simulink model "Fig_11_12_13_"  (R2024a)
settings: Solver=VariableStepAuto  StartTime=0.0  StopTime=1  RelTol=1e-3
undefined symbols (not defined in the file): gcbh, Ion, Lithium, sps_rtmsupport
libraries: spsSeriesRLCBranchLib x11, slpidlib x5, spsIGBTDiodeLib x4, spsVoltageMeasurementLib x4, spsThreePhaseVIMeasurementLib x4, spsThreePhaseSeriesRLCBranchLib x4, spsUniversalBridgeLib x3, spsPWMGeneratorDCDCLib x3, spsVIMeasurementModel x3, spsDiodeLib x2, spsabctodq0Lib x2, spsCurrentMeasurementLib x2
(part 1 of 2)
settings Model: Creator=MS  LastModifiedBy=Dileep Uppara
settings DataIOCC: ReturnWorkspaceOutputs=off

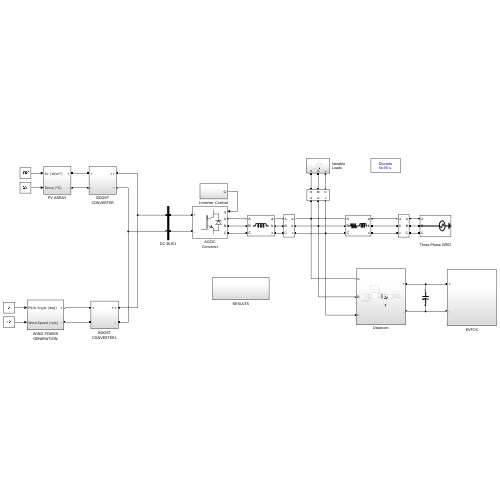
[thumbnail: Simulink's stored preview of the top-level diagram]
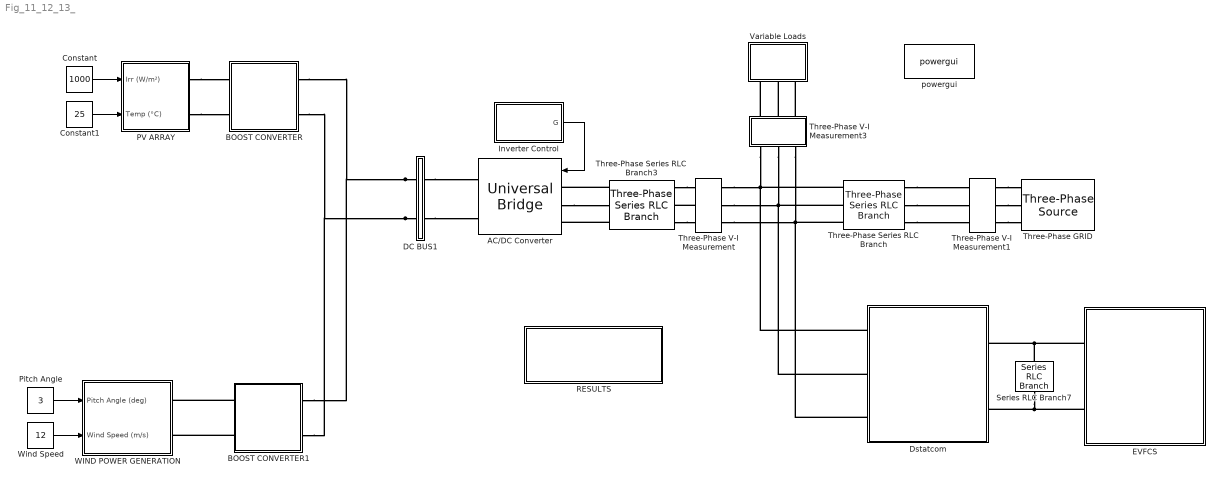
== system Fig_11_12_13_ ==
  " Three-Phase GRID" : spsThreePhaseSourceLib/Three-Phase Source  InternalConnection=Yg  VoltagePhases=off  Voltage=400  PhaseAngle=0  Voltage_phases=[25e3 25e3 25e3]/sqrt(3)  PhaseAngles_phases=[0 -120 +120]  Frequency=50  NonIdealSource=on  SpecifyImpedance=off  Resistance=0  Inductance=0  ShortCircuitLevel=100e6  BaseVoltage=0  XRratio=7  BusType=swing  Pref=0  Qref=0  Prefabc=[10e3, 10e3, 10e3]  Qrefabc=[0, 0, 0]  Qmin=-inf  Qmax=inf
  AC/DC Converter : spsUniversalBridgeLib/Universal Bridge  Arms=3  SnubberResistance=1e5  SnubberCapacitance=inf  Device=IGBT / Diodes  Ron=1e-3  Lon=0  ForwardVoltages="[  0  0  ]"  ForwardVoltage=0  GTOparameters=[ 10e-6 , 20e-6 ]  IGBTparameters=[ 1e-6 , 2e-6 ]  Measurements=None  Measurements_2=None  converterType=Rectifier
  BOOST CONVERTER : Subsystem
  BOOST CONVERTER1 : Subsystem
  Constant : Constant  Value=1000  SampleTime=50e-6
  Constant1 : Constant  Value=25  SampleTime=50e-6
  DC BUS1 : Subsystem
  Dstatcom : Subsystem
  EVFCS : Subsystem
  Inverter Control : Subsystem
  PV ARRAY : Subsystem
  "Pitch Angle " : Constant  Value=3  SampleTime=50e-6
  RESULTS : Subsystem
  Series RLC Branch7 : spsSeriesRLCBranchLib/Series RLC Branch  LConnTagsString=__new0  RConnTagsString=__new0  BranchType=C  Resistance=1  Inductance=1e-3  SetiL0=off  InitialCurrent=0  Capacitance=1000e-6  Setx0=on  InitialVoltage=800  Measurements=None
  Three-Phase Series RLC Branch : spsThreePhaseSeriesRLCBranchLib/Three-Phase Series RLC Branch  LConnTagsString=A|B|C  RConnTagsString=A|B|C  BranchType=RL  Resistance=2.088  Inductance=0.01e-3  Capacitance=1e-6  Measurements=None
  Three-Phase Series RLC Branch3 : spsThreePhaseSeriesRLCBranchLib/Three-Phase Series RLC Branch  LConnTagsString=A|B|C  RConnTagsString=A|B|C  BranchType=L  Resistance=3  Inductance=20e-3  Capacitance=1e-6  Measurements=None
  Three-Phase V-I Measurement : spsThreePhaseVIMeasurementLib/Three-Phase V-I Measurement  VoltageMeasurement=phase-to-ground  SetLabelV=on  LabelV=Viabc  Vpu=off  VpuLL=off  CurrentMeasurement=yes  SetLabelI=on  LabelI=Iiabc  Ipu=off  Pbase=100e6  Vbase=500e3  OutputType=Complex  PhasorSimulation=off  PSBequivalent=0
  Three-Phase V-I Measurement1 : spsThreePhaseVIMeasurementLib/Three-Phase V-I Measurement  VoltageMeasurement=phase-to-ground  SetLabelV=on  LabelV=Vgabc  Vpu=off  VpuLL=off  CurrentMeasurement=yes  SetLabelI=on  LabelI=Igabc  Ipu=off  Pbase=100e6  Vbase=500e3  OutputType=Complex  PhasorSimulation=off  PSBequivalent=0
  Three-Phase V-I Measurement3 : Subsystem  DialogController=POWERSYS.PowerSysDialog  LoadFcn=|  StartFcn=sps_rtmsupport('StartFcn',gcbh);  StopFcn=sps_rtmsupport('StopFcn',gcbh);  mask(Three-Phase VI Measurement){VoltageMeasurement=phase-to-ground, SetLabelV=on, LabelV=Vlabc, Vpu=off, VpuLL=off, CurrentMeasurement=yes, SetLabelI=on, LabelI=Ilabc, Ipu=off, Pbase=100e6, Vbase=500e3, OutputType=Complex, PhasorSimulation=off, PSBequivalent=0}
      | if ~strcmp(get_param(bdroot,'BlockDiagramType'),'library')
      |     set_param([gcb,'/Model'],'LinkStatus','restore');
      | end
      | sps_rtmsupport('LoadFcn',gcbh);
      mask prompts: VoltageMeasurement "Voltage measurement"; SetLabelV "Use a label"; LabelV "Signal label  (use a From block to collect this signal)"; Vpu "Voltages in pu,  based on peak value of nominal phase-to-ground voltage"; VpuLL "Voltages in pu,  based on peak value of nominal phase-to-phase  voltage"; CurrentMeasurement "Current measurement"; SetLabelI "Use a label"; LabelI "Signal label  (use a From block to collect this signal)"; Ipu "Currents in pu"; Pbase "Base power ( VA 3 phase)"; Vbase "Nominal voltage used for pu measurement (Vrms phase-phase) :"; OutputType "Output signals in:"; PhasorSimulation "Phasor simulation (internal use)"; PSBequivalent "Equivalent circuit (internal use)"
      mask help:
      | Ideal three-phase voltage and current measurements.
      |
      | The block can output the voltages and currents in per unit values or in volts and amperes.
      mask init:
      | block = gcb;
      | Kv=1;
      | Ki=1;
      | [Kv,Ki] = powericon('ThreePhaseVIMeasurementParam',block,Vpu,VpuLL,Ipu,Vbase,Pbase,PhasorSimulation,OutputType);
      | powericon('ThreePhaseVIMeasurementCback',block);
      | power_initmask();
      settings: CopyFcn=sps_rtmsupport('CopyFcn',gcbh); powericon('ThreePhaseVIMeasurementCopy',gcb)  DeleteFcn=sps_rtmsupport('DeleteFcn',gcbh);  UndoDeleteFcn=sps_rtmsupport('UndoDeleteFcn',gcbh);  ModelCloseFcn=sps_rtmsupport('ModelCloseFcn',gcbh);  PostSaveFcn=sps_rtmsupport('PostSaveFcn',gcbh);  NameChangeFcn=sps_rtmsupport('NameChangeFcn',gcbh);  PreCopyFcn=sps_rtmsupport('PreCopyFcn',gcbh);  OpenFcn=sps_rtmsupport('OpenFcn',gcbh, [1 2 4 5 6 7 9 -12 13]);  CloseFcn=sps_rtmsupport('CloseFcn',gcbh);  PreDeleteFcn=sps_rtmsupport('PreDeleteFcn',gcbh);
      settings: LibrarySourceBlock=|
      | sps_lib/Sensors and Measurements/Three-Phase
      | V-I Measurement
      settings: PreSaveFcn=|
      | sps_rtmsupport('PreSaveFcn',gcbh);
      | if ~strcmp(get_param(bdroot(gcbh),'BlockDiagramType'),'library')
      |     set_param(gcb,'LinkStatus','restore')
      | end
      mask Help: helpview(psbhelp)
      mask TypeOptions VoltageMeasurement: no | phase-to-ground | phase-to-phase
      mask Callback VoltageMeasurement: powericon('ThreePhaseVIMeasurementCback',gcb,'Vselector');
      mask Callback SetLabelV: powericon('ThreePhaseVIMeasurementCback',gcb,'');
      mask Callback Vpu: powericon('ThreePhaseVIMeasurementCback',gcb,'Vpu');
      mask Callback VpuLL: powericon('ThreePhaseVIMeasurementCback',gcb,'VpuLL');
      mask TypeOptions CurrentMeasurement: no | yes
      mask Callback CurrentMeasurement: powericon('ThreePhaseVIMeasurementCback',gcb,'');
      mask Callback SetLabelI: powericon('ThreePhaseVIMeasurementCback',gcb,'');
      mask Callback LabelI: powericon('ThreePhaseVIMeasurementCback',gcb,'');
      mask Callback Ipu: powericon('ThreePhaseVIMeasurementCback',gcb,'');
      mask TypeOptions OutputType: Complex | Real-Imag | Magnitude-Angle | Magnitude
  Variable Loads : Subsystem
  WIND POWER GENERATION : Subsystem
  Wind Speed : Constant  Value=12  SampleTime=50e-6
  powergui : spspowerguiLib/powergui  Priority=1  SimulationMode=Discrete  SampleTime=50e-6  frequency=60  Iterations=50  frequencyindice=0  Pbase=100e6  ErrMax=1e-4  UnitsV=kV  UnitsW=MW  buscounter=0  FunctionMessages=off  echomessages=off  EnableUseOfTLC=off  CurrentSourceSwitches=off  DisableSnubberDevices=off  DisableRonSwitches=off  DisableVfSwitches=off  DisplayEquations=off  AutomaticDiscreteSolvers=off  SolverType=Tustin/Backward Euler (TBE)  Interpol=off  ExternalGateDelay=off  methode=off  Ts=100  x0status=blocks  SPID=on  SwTol=0  HookPort=off  NonlinearTolerance=1e-4  nMaxIteration=100  ContinueOnMaxIteration=off  RestoreLinks=warning  ResistiveCurrentMeasurement=off  Frange=[0:2:500]  Ylog=off  Xlog=on  ShowGrid=off  save=off  variable=ZData  structure=0  ZoomFFT=off  StartTime=0.0  cycles=1  DisplayStyle=1  fundamental=60  FreqAxis=off  MaxFrequency=1000  frequencyindicesteady=1  RmsSteady=1  display=off
  wires:
  Inverter Control/1(G) -> AC/DC Converter/1
  Wind Speed/1 -> WIND POWER GENERATION/2(Wind Speed (m/s))
  "Pitch Angle "/1 -> WIND POWER GENERATION/1(Pitch Angle (deg))
  Constant/1 -> PV ARRAY/1(Irr (W/m²))
  Constant1/1 -> PV ARRAY/2(Temp (°C))
  connections:
  Three-Phase Series RLC Branch3/LConn1 -- AC/DC Converter/LConn1
  AC/DC Converter/LConn2 -- Three-Phase Series RLC Branch3/LConn2
  Three-Phase Series RLC Branch3/LConn3 -- AC/DC Converter/LConn3
  Three-Phase Series RLC Branch3/RConn1 -- Three-Phase V-I Measurement/LConn1
  Three-Phase V-I Measurement/LConn2 -- Three-Phase Series RLC Branch3/RConn2
  Three-Phase Series RLC Branch3/RConn3 -- Three-Phase V-I Measurement/LConn3
  DC BUS1/RConn2 -- AC/DC Converter/RConn2
  DC BUS1/RConn1 -- AC/DC Converter/RConn1
  Three-Phase V-I Measurement/RConn1 -- Three-Phase V-I Measurement3/RConn1 -- Three-Phase Series RLC Branch/LConn1 -- Dstatcom/RConn1
  Three-Phase V-I Measurement/RConn3 -- Three-Phase V-I Measurement3/RConn3 -- Three-Phase Series RLC Branch/LConn3 -- Dstatcom/RConn3
  Three-Phase V-I Measurement/RConn2 -- Three-Phase V-I Measurement3/RConn2 -- Three-Phase Series RLC Branch/LConn2 -- Dstatcom/RConn2
  Series RLC Branch7/LConn1 -- EVFCS/RConn1 -- Dstatcom/LConn1
  Series RLC Branch7/RConn1 -- Dstatcom/LConn2 -- EVFCS/RConn2
  DC BUS1/LConn2 -- BOOST CONVERTER/RConn2 -- BOOST CONVERTER1/RConn2
  DC BUS1/LConn1 -- BOOST CONVERTER/RConn1 -- BOOST CONVERTER1/RConn1
  Three-Phase V-I Measurement3/LConn2 -- Variable Loads/LConn2
  Three-Phase V-I Measurement3/LConn1 -- Variable Loads/LConn1
  Three-Phase V-I Measurement3/LConn3 -- Variable Loads/LConn3
  PV ARRAY/RConn1 -- BOOST CONVERTER/LConn1
  PV ARRAY/RConn2 -- BOOST CONVERTER/LConn2
  BOOST CONVERTER1/LConn2 -- WIND POWER GENERATION/RConn2
  BOOST CONVERTER1/LConn1 -- WIND POWER GENERATION/RConn1
  Three-Phase V-I Measurement1/LConn1 -- " Three-Phase GRID"/RConn1
  Three-Phase Series RLC Branch/RConn2 -- Three-Phase V-I Measurement1/RConn2
  Three-Phase V-I Measurement1/LConn3 -- " Three-Phase GRID"/RConn3
  Three-Phase Series RLC Branch/RConn1 -- Three-Phase V-I Measurement1/RConn1
  Three-Phase V-I Measurement1/LConn2 -- " Three-Phase GRID"/RConn2
  Three-Phase Series RLC Branch/RConn3 -- Three-Phase V-I Measurement1/RConn3

== system Fig_11_12_13_/BOOST CONVERTER ==
  Diode : spsDiodeLib/Diode  Ron=0.001  Lon=0  Vf=0.8  IC=0  UseSnubber=0  Rs=500  Cs=250e-9  Measurements=off
  IGBT/Diode : spsIGBTDiodeLib/IGBT//Diode  Ron=1e-3  Rs=1e5  Cs=inf  Measurements=off
  PWM Generator (DC-DC) : spsPWMGeneratorDCDCLib/PWM Generator (DC-DC)  Fsw=15e3  Ts=50e-6
  PnO : Subsystem
  Series RLC Branch : spsSeriesRLCBranchLib/Series RLC Branch  LConnTagsString=__new0  RConnTagsString=__new0  BranchType=L  Resistance=0.01  Inductance=0.009e-3  SetiL0=off  InitialCurrent=0  Capacitance=1e-6  Setx0=off  InitialVoltage=0  Measurements=None
  Series RLC Branch1 : spsSeriesRLCBranchLib/Series RLC Branch  LConnTagsString=__new0  RConnTagsString=__new0  BranchType=C  Resistance=0.01  Inductance=0.5e-3  SetiL0=off  InitialCurrent=0  Capacitance=880e-6  Setx0=off  InitialVoltage=0  Measurements=None
  Series RLC Branch2 : spsSeriesRLCBranchLib/Series RLC Branch  LConnTagsString=__new0  RConnTagsString=__new0  BranchType=C  Resistance=0.01  Inductance=0.5e-3  SetiL0=off  InitialCurrent=0  Capacitance=880e-6  Setx0=off  InitialVoltage=0  Measurements=None
  + : PMIOPort  Side=Left
  - : PMIOPort  Port=2  Side=Left
  ++ : PMIOPort  Port=3  Side=Right
  -- : PMIOPort  Port=4  Side=Right
  wires:
  PWM Generator (DC-DC)/1 -> IGBT/Diode/1
  PnO/1(D) -> PWM Generator (DC-DC)/1
  connections:
  Series RLC Branch/RConn1 -- Diode/LConn1 -- IGBT/Diode/LConn1
  +/RConn1 -- Series RLC Branch2/LConn1 -- Series RLC Branch/LConn1
  Series RLC Branch2/RConn1 -- -/RConn1 -- Series RLC Branch1/RConn1 -- --/RConn1 -- IGBT/Diode/RConn1
  Diode/RConn1 -- ++/RConn1 -- Series RLC Branch1/LConn1

== system Fig_11_12_13_/BOOST CONVERTER1 ==
  Diode : spsDiodeLib/Diode  Ron=0.001  Lon=0  Vf=0.8  IC=0  UseSnubber=0  Rs=500  Cs=250e-9  Measurements=off
  IGBT/Diode : spsIGBTDiodeLib/IGBT//Diode  Ron=1e-3  Rs=1e5  Cs=inf  Measurements=off
  PWM Generator (DC-DC) : spsPWMGeneratorDCDCLib/PWM Generator (DC-DC)  Fsw=15e3  Ts=50e-6
  PnO : Subsystem
  Series RLC Branch : spsSeriesRLCBranchLib/Series RLC Branch  LConnTagsString=__new0  RConnTagsString=__new0  BranchType=RL  Resistance=1.524  Inductance=0.1e-3  SetiL0=off  InitialCurrent=0  Capacitance=1e-6  Setx0=off  InitialVoltage=0  Measurements=None
  Series RLC Branch1 : spsSeriesRLCBranchLib/Series RLC Branch  LConnTagsString=__new0  RConnTagsString=__new0  BranchType=C  Resistance=0.01  Inductance=0.5e-3  SetiL0=off  InitialCurrent=0  Capacitance=880e-6  Setx0=off  InitialVoltage=0  Measurements=None
  + : PMIOPort  Side=Left
  - : PMIOPort  Port=2  Side=Left
  ++ : PMIOPort  Port=3  Side=Right
  -- : PMIOPort  Port=4  Side=Right
  wires:
  PWM Generator (DC-DC)/1 -> IGBT/Diode/1
  PnO/1(D) -> PWM Generator (DC-DC)/1
  connections:
  Series RLC Branch/RConn1 -- Diode/LConn1 -- IGBT/Diode/LConn1
  Diode/RConn1 -- Series RLC Branch1/LConn1 -- ++/RConn1
  +/RConn1 -- Series RLC Branch/LConn1
  -/RConn1 -- Series RLC Branch1/RConn1 -- --/RConn1 -- IGBT/Diode/RConn1

== system Fig_11_12_13_/DC BUS1 ==
  Display5 : Display
  Scope5 : Scope
  Series RLC Branch1 : spsSeriesRLCBranchLib/Series RLC Branch  LConnTagsString=__new0  RConnTagsString=__new0  BranchType=C  Resistance=0.01  Inductance=0.5e-3  SetiL0=off  InitialCurrent=0  Capacitance=10000e-6  Setx0=off  InitialVoltage=0  Measurements=None
  Voltage Measurement1 : spsVoltageMeasurementLib/Voltage Measurement  PhasorSimulation=off  OutputType=Complex  PSBequivalent=0
  ++ : PMIOPort  Side=Left
  Connection Port1 : PMIOPort  Port=2  Side=Left
  + : PMIOPort  Port=3  Side=Right
  - : PMIOPort  Port=4  Side=Right
  tag scope: Vdc=global
  wires:
  Voltage Measurement1/1 -> [Vdc], Display5/1, Scope5/1
  connections:
  -/RConn1 -- Voltage Measurement1/LConn2 -- Series RLC Branch1/RConn1 -- Connection Port1/RConn1
  +/RConn1 -- Series RLC Branch1/LConn1 -- ++/RConn1 -- Voltage Measurement1/LConn1

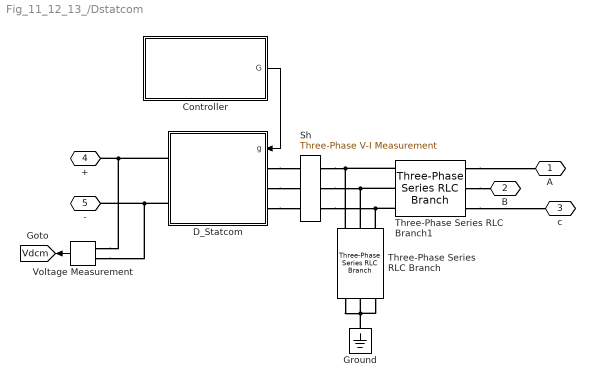
== system Fig_11_12_13_/Dstatcom ==
  Controller : Subsystem
  D_Statcom : Subsystem  DialogController=POWERSYS.PowerSysDialog  LoadFcn=sps_rtmsupport('LoadFcn',gcbh);  StartFcn=sps_rtmsupport('StartFcn',gcbh);  StopFcn=sps_rtmsupport('StopFcn',gcbh);  mask(Universal Bridge){Arms=3, SnubberResistance=1e5, SnubberCapacitance=inf, Device=IGBT / Diodes, Ron=1e-3, Lon=0, ForwardVoltages=[  0  0  ], ForwardVoltage=0, GTOparameters=[ 10e-6 , 20e-6 ], IGBTparameters=[ 1e-6 , 2e-6 ], Measurements=None, Measurements_2=None, converterType=Rectifier}
      mask prompts: Arms "Number of bridge arms:"; SnubberResistance "Snubber resistance Rs (Ohms)"; SnubberCapacitance "Snubber capacitance Cs (F)"; Device "Power Electronic device"; Ron "Ron (Ohms)"; Lon "Lon (H)"; ForwardVoltages "Forward voltages  [ Device Vf(V) , Diode Vfd(V)]"; ForwardVoltage "Forward voltage Vf (V)"; GTOparameters "[  Tf (s) , Tt (s)  ]"; IGBTparameters "[  Tf (s) , Tt (s)  ]"; Measurements_2 "Measurements"; converterType "Converter type:"
      mask help: This block implement a bridge of selected power electronics devices. Series RC snubber circuits are connected in parallel with each switch device. Press Help for suggested snubber values when the model is discretized. For most applications the internal inductance Lon of diodes and thyristors should be set to zero
      mask init:
      | block = gcb;
      | [WantBlockChoice,Ts,Switches,Tf_sps,Tt_sps,Vf,Vf_SwitchOn,Vf_DiodeOn,IC,SignalLength,ReorderGatesDelays,X,Y,Ron] = powericon('UniversalBridgeInit',block,Device,Arms,ForwardVoltage,ForwardVoltages,GTOparameters,IGBTparameters,Ron);
      | powericon('SetInternalModels','set',block,WantBlockChoice);
      settings: LibrarySourceBlock=sps_lib/Power Electronics/Universal Bridge  CopyFcn=sps_rtmsupport('CopyFcn',gcbh); powericon('SwitchesCopyFcn','Universal Bridge',gcb)  DeleteFcn=sps_rtmsupport('DeleteFcn',gcbh);  UndoDeleteFcn=sps_rtmsupport('UndoDeleteFcn',gcbh);  ModelCloseFcn=sps_rtmsupport('ModelCloseFcn',gcbh);  PreSaveFcn=sps_rtmsupport('PreSaveFcn',gcbh);  PostSaveFcn=sps_rtmsupport('PostSaveFcn',gcbh);  NameChangeFcn=sps_rtmsupport('NameChangeFcn',gcbh);  PreCopyFcn=sps_rtmsupport('PreCopyFcn',gcbh);  OpenFcn=sps_rtmsupport('OpenFcn',gcbh, [1 4 11 12 13]);  CloseFcn=sps_rtmsupport('CloseFcn',gcbh);  PreDeleteFcn=sps_rtmsupport('PreDeleteFcn',gcbh);
      mask Help: helpview(psbhelp);
      mask TypeOptions Arms: 1 | 2 | 3
      mask Callback Arms: powericon('UniversalBridgeCback',gcb);
      mask TypeOptions Device: Diodes | Thyristors | GTO / Diodes | MOSFET / Diodes | IGBT / Diodes | Ideal Switches | Switching-function based VSC | Average-model based VSC
      mask Callback Device: powericon('UniversalBridgeCback',gcb);
      mask TypeOptions Measurements: None | Device voltages | Device currents | UAB UBC UCA UDC voltages | All voltages and currents
      mask TypeOptions Measurements_2: None | Voltages | Currents | Voltages and Currents
      mask TypeOptions converterType: Rectifier | Inverter
      mask Display: plot(0,0,100,100,X.p1,Y.p1,X.p2,Y.p2,X.p3,Y.p3,X.p4,Y.p4,X.p5,Y.p5,X.p6,Y.p6,X.p7,Y.p7);
  Ground : spsGroundLib/Ground  LConnTagsString=a
  Sh : spsThreePhaseVIMeasurementLib/Three-Phase V-I Measurement  VoltageMeasurement=phase-to-ground  SetLabelV=on  LabelV=Vshabc  Vpu=off  VpuLL=off  CurrentMeasurement=yes  SetLabelI=on  LabelI=Ishabc  Ipu=off  Pbase=100e6  Vbase=500e3  OutputType=Complex  PhasorSimulation=off  PSBequivalent=0
  Three-Phase Series RLC Branch : spsThreePhaseSeriesRLCBranchLib/Three-Phase Series RLC Branch  LConnTagsString=A|B|C  RConnTagsString=A|B|C  BranchType=C  Resistance=1  Inductance=1e-3  Capacitance=220e-6  Measurements=None
  Three-Phase Series RLC Branch1 : spsThreePhaseSeriesRLCBranchLib/Three-Phase Series RLC Branch  LConnTagsString=A|B|C  RConnTagsString=A|B|C  BranchType=RL  Resistance=0.1  Inductance=1e-3  Capacitance=1e-6  Measurements=None
  Voltage Measurement : spsVoltageMeasurementLib/Voltage Measurement  PhasorSimulation=off  OutputType=Complex  PSBequivalent=0
  A : PMIOPort  Side=Right
  B : PMIOPort  Port=2  Side=Right
  "c " : PMIOPort  Port=3  Side=Right
  + : PMIOPort  Port=4  Side=Left
  - : PMIOPort  Port=5  Side=Left
  tag scope: Vdcm=global
  wires:
  Voltage Measurement/1 -> [Vdcm]
  Controller/1(G) -> D_Statcom/1(g)
  connections:
  Sh/RConn2 -- Three-Phase Series RLC Branch1/LConn2 -- Three-Phase Series RLC Branch/LConn2
  Three-Phase Series RLC Branch1/RConn3 -- "c "/RConn1
  Three-Phase Series RLC Branch1/RConn2 -- B/RConn1
  Sh/RConn1 -- Three-Phase Series RLC Branch1/LConn1 -- Three-Phase Series RLC Branch/LConn1
  Three-Phase Series RLC Branch1/RConn1 -- A/RConn1
  Sh/RConn3 -- Three-Phase Series RLC Branch1/LConn3 -- Three-Phase Series RLC Branch/LConn3
  Ground/LConn1 -- Three-Phase Series RLC Branch/RConn3 -- Three-Phase Series RLC Branch/RConn1 -- Three-Phase Series RLC Branch/RConn2
  D_Statcom/RConn1 -- Voltage Measurement/LConn1 -- +/RConn1
  D_Statcom/RConn2 -- -/RConn1 -- Voltage Measurement/LConn2
  D_Statcom/LConn3 -- Sh/LConn3
  D_Statcom/LConn2 -- Sh/LConn2
  D_Statcom/LConn1 -- Sh/LConn1

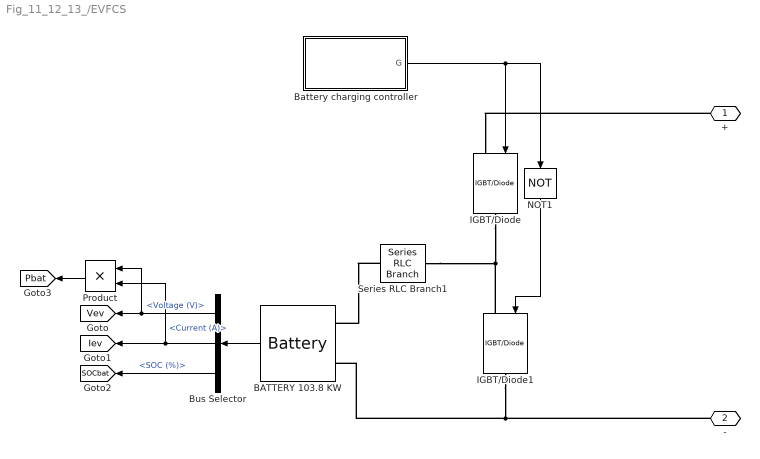
== system Fig_11_12_13_/EVFCS ==
  BATTERY 103.8 KW : spsBatteryLib/Battery  BatType=Lithium-Ion  ShowTempParam=off  ThermalPreset=no  ShowAgeParam=off  NomV=480  NomQ=100  SOC=60  Batt_Tr=1e-3  PresetModel=on  MaxQ=100  MinV=360  FullV=558.7138  Dis_rate=43.4783  R=0.048  Normal_OP=90.4348  expZone="[518.5852      4.913043]"  current=[6.5 13 32.5]  Units=Time  Tci=20  NomT=20  T2=-30  MaxQ2=4.8  FullV2=7.1  Normal_OP2=5.655  expZone2="[6.58           1]"  Rca=0.6  ti=2000  Dp=0  Neq0=0  Tsim=1e6  Ta1=25  Qeol=5.4*0.9  Reol=0.013333*1.2  Char_age=[2.3478, 3]  Dis_age=[2.3478, 10]  N1=1500  N2=10500  N3=1000  N4=1400  Ta2=45  N5=950
  Battery charging controller : Subsystem
  Bus Selector : BusSelector  OutputSignals=Voltage (V),Current (A),SOC (%)
  IGBT/Diode : spsIGBTDiodeLib/IGBT//Diode  Ron=1e-3  Rs=1e5  Cs=inf  Measurements=off
  IGBT/Diode1 : spsIGBTDiodeLib/IGBT//Diode  Ron=1e-3  Rs=1e5  Cs=inf  Measurements=off
  NOT1 : Logic  Operator=NOT  IconShape=distinctive  AllPortsSameDT=off  OutDataTypeStr=boolean
  Product : Product
  Series RLC Branch1 : spsSeriesRLCBranchLib/Series RLC Branch  LConnTagsString=__new0  RConnTagsString=__new0  BranchType=RL  Resistance=5.1  Inductance=100e-3  SetiL0=off  InitialCurrent=0  Capacitance=1e-6  Setx0=off  InitialVoltage=0  Measurements=None
  + : PMIOPort  Side=Right
  - : PMIOPort  Port=2  Side=Right
  tag scope: Iev=global, Pbat=global, SOCbat=global, Vev=global
  wires:
  Bus Selector/3 -> [SOCbat]  "<SOC (%)>"
  Bus Selector/2 -> Product/2, [Iev]  "<Current (A)>"
  Bus Selector/1 -> Product/1, [Vev]  "<Voltage (V)>"
  BATTERY 103.8 KW/1 -> Bus Selector/1
  Product/1 -> [Pbat]
  Battery charging controller/1(G) -> IGBT/Diode/1, NOT1/1
  NOT1/1 -> IGBT/Diode1/1
  connections:
  Series RLC Branch1/LConn1 -- BATTERY 103.8 KW/LConn1
  IGBT/Diode/RConn1 -- Series RLC Branch1/RConn1 -- IGBT/Diode1/LConn1
  +/RConn1 -- IGBT/Diode/LConn1
  IGBT/Diode1/RConn1 -- -/RConn1 -- BATTERY 103.8 KW/LConn2

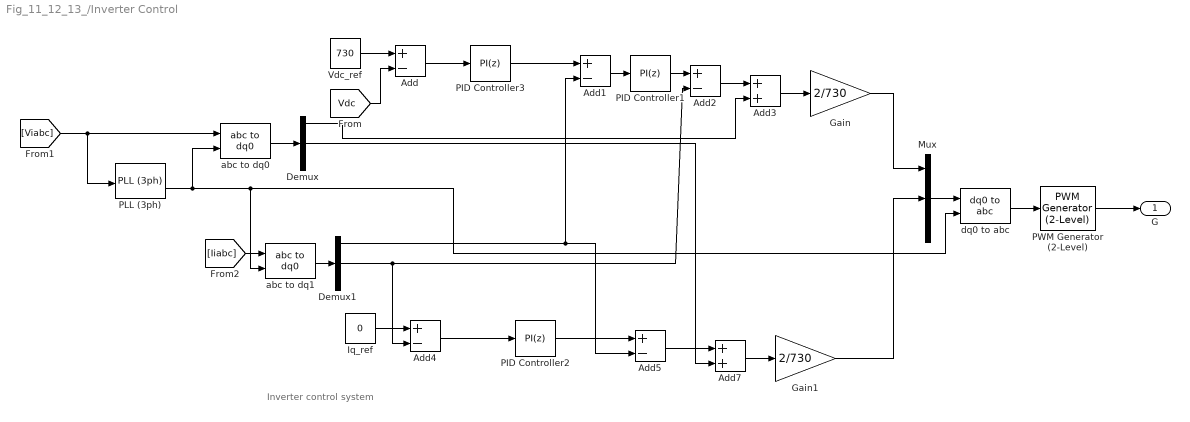
== system Fig_11_12_13_/Inverter Control ==
  note: Inverter control system
  Add{,1..2,4..5} (5 alike) : Sum  Inputs=+-
  Add3 : Sum
  Add7 : Sum
  Demux : Demux  Outputs=3
  Demux1 : Demux  Outputs=3
  Gain : Gain  Gain=2/730
  Gain1 : Gain  Gain=2/730
  Iq_ref : Constant  Value=0
  Mux : Mux  Inputs=3
  PID Controller1 : slpidlib/PID Controller  Controller=PI  Form=Parallel  TimeDomain=Discrete-time  UseExternalTs=off  SampleTime=-1  IntegratorMethod=Forward Euler  FilterMethod=Forward Euler  ControllerParametersSource=internal  P=0.5  I=200  UseKiTs=off  D=0  UseExternalDerivativeSource=off  N=100  UseFilter=on  TunerSelectOption=Transfer Function Based (PID Tuner App)  InitialConditionSource=internal  InitialConditionForIntegrator=0  InitialConditionForFilter=0  DifferentiatorICPrevScaledInput=0  ExternalReset=none  TrackingMode=off  Kt=1  LimitOutput=off  SatLimitsSource=internal  UpperSaturationLimit=inf  LowerSaturationLimit=-inf  LinearizeAsGain=on  AntiWindupMode=none  Kb=1  LimitIntegrator=off  UpperIntegratorSaturationLimit=inf  LowerIntegratorSaturationLimit=-inf  POutMin=[]  POutMax=[]  IOutMin=[]  IOutMax=[]  DOutMin=[]  DOutMax=[]  NOutMin=[]  NOutMax=[]  SumOutMin=[]  SumOutMax=[]  SaturationOutMin=[]  SaturationOutMax=[]  PParamMin=[]  PParamMax=[]  IParamMin=[]  IParamMax=[]  DParamMin=[]  DParamMax=[]  NParamMin=[]  NParamMax=[]  KbParamMin=[]  KbParamMax=[]  KtParamMin=[]  KtParamMax=[]  KbOutMin=[]  KbOutMax=[]  KtOutMin=[]  KtOutMax=[]  IntegratorOutMin=[]  IntegratorOutMax=[]  FilterOutMin=[]  FilterOutMax=[]  SumI1OutMin=[]  SumI1OutMax=[]  SumI2OutMin=[]  SumI2OutMax=[]  SumI3OutMin=[]  SumI3OutMax=[]  SumI4OutMin=[]  SumI4OutMax=[]  SumDOutMin=[]  SumDOutMax=[]  DifferentiatorOutMin=[]  DifferentiatorOutMax=[]  FilterDiffOutCoefMin=[]  FilterDiffOutCoefMax=[]  ReciprocalOutMin=[]  ReciprocalOutMax=[]  SumDenOutMin=[]  SumDenOutMax=[]  SumNumOutMin=[]  SumNumOutMax=[]  DivideOutMin=[]  DivideOutMax=[]  UdiffTsProdOutMin=[]  UdiffTsProdOutMax=[]  NTsProdOutMin=[]  NTsProdOutMax=[]  UintegralTsProdOutMin=[]  UintegralTsProdOutMax=[]  UngainTsProdOutMin=[]  UngainTsProdOutMax=[]  ClampingZeroOutDataTypeStr=Inherit: Inherit via back propagation  ClampingZeroOutMin=[]  ClampingZeroOutMax=[]  FilterDenConstantOutDataTypeStr=Inherit: Inherit via back propagation  FilterDenConstantOutMin=[]  FilterDenConstantOutMax=[]  PCopyOutDataTypeStr=Inherit: Inherit via back propagation  PCopyOutMin=[]  PCopyOutMax=[]  NCopyOutDataTypeStr=Inherit: Inherit via back propagation  NCopyOutMin=[]  NCopyOutMax=[]  IntegratorContinuousStateAttributes=''  IntegratorStateMustResolveToSignalObject=off  IntegratorRTWStateStorageClass=Auto  FilterContinuousStateAttributes=''  FilterStateMustResolveToSignalObject=off  FilterRTWStateStorageClass=Auto  ParallelPVariant=InternalParameters  IdealPVariant=Disabled  IVariant=InternalParameters  DVariant=Disabled  IntegratorVariant=Discrete  SatVariant=Disabled  AWVariant=Passthrough  PCopyVariant=Disabled  TRVariant=Disabled  FdbkBlocksVariant=Forward  IdealPFdbkVariant=Disabled  SatFdbkVariant=Disabled  DerivativeFilterVariant=Disabled  NVariant=Disabled  NCopyVariant=Disabled_SignalSpec  FilterICVariant=Disabled  IntegratorICVariant=InternalICs  ExternalResetVariant=Disabled  TRSumVariant=Passthrough  SumFdbkVariant=Disabled  SumVariant=Sum_PI  TsampFilterVariant=InternalTs  TsampNgainVariant=Passthrough  TsampIntegralVariant=Disabled_SignalSpec  ExternalSaturationOutDataTypeStr=Inherit: Same as second input  DerivativeSourceVariant=Disabled
  PID Controller2 : slpidlib/PID Controller  Controller=PI  Form=Parallel  TimeDomain=Discrete-time  UseExternalTs=off  SampleTime=-1  IntegratorMethod=Forward Euler  FilterMethod=Forward Euler  ControllerParametersSource=internal  P=0.5  I=200  UseKiTs=off  D=0  UseExternalDerivativeSource=off  N=100  UseFilter=on  TunerSelectOption=Transfer Function Based (PID Tuner App)  InitialConditionSource=internal  InitialConditionForIntegrator=0  InitialConditionForFilter=0  DifferentiatorICPrevScaledInput=0  ExternalReset=none  TrackingMode=off  Kt=1  LimitOutput=off  SatLimitsSource=internal  UpperSaturationLimit=inf  LowerSaturationLimit=-inf  LinearizeAsGain=on  AntiWindupMode=none  Kb=1  LimitIntegrator=off  UpperIntegratorSaturationLimit=inf  LowerIntegratorSaturationLimit=-inf  POutMin=[]  POutMax=[]  IOutMin=[]  IOutMax=[]  DOutMin=[]  DOutMax=[]  NOutMin=[]  NOutMax=[]  SumOutMin=[]  SumOutMax=[]  SaturationOutMin=[]  SaturationOutMax=[]  PParamMin=[]  PParamMax=[]  IParamMin=[]  IParamMax=[]  DParamMin=[]  DParamMax=[]  NParamMin=[]  NParamMax=[]  KbParamMin=[]  KbParamMax=[]  KtParamMin=[]  KtParamMax=[]  KbOutMin=[]  KbOutMax=[]  KtOutMin=[]  KtOutMax=[]  IntegratorOutMin=[]  IntegratorOutMax=[]  FilterOutMin=[]  FilterOutMax=[]  SumI1OutMin=[]  SumI1OutMax=[]  SumI2OutMin=[]  SumI2OutMax=[]  SumI3OutMin=[]  SumI3OutMax=[]  SumI4OutMin=[]  SumI4OutMax=[]  SumDOutMin=[]  SumDOutMax=[]  DifferentiatorOutMin=[]  DifferentiatorOutMax=[]  FilterDiffOutCoefMin=[]  FilterDiffOutCoefMax=[]  ReciprocalOutMin=[]  ReciprocalOutMax=[]  SumDenOutMin=[]  SumDenOutMax=[]  SumNumOutMin=[]  SumNumOutMax=[]  DivideOutMin=[]  DivideOutMax=[]  UdiffTsProdOutMin=[]  UdiffTsProdOutMax=[]  NTsProdOutMin=[]  NTsProdOutMax=[]  UintegralTsProdOutMin=[]  UintegralTsProdOutMax=[]  UngainTsProdOutMin=[]  UngainTsProdOutMax=[]  ClampingZeroOutDataTypeStr=Inherit: Inherit via back propagation  ClampingZeroOutMin=[]  ClampingZeroOutMax=[]  FilterDenConstantOutDataTypeStr=Inherit: Inherit via back propagation  FilterDenConstantOutMin=[]  FilterDenConstantOutMax=[]  PCopyOutDataTypeStr=Inherit: Inherit via back propagation  PCopyOutMin=[]  PCopyOutMax=[]  NCopyOutDataTypeStr=Inherit: Inherit via back propagation  NCopyOutMin=[]  NCopyOutMax=[]  IntegratorContinuousStateAttributes=''  IntegratorStateMustResolveToSignalObject=off  IntegratorRTWStateStorageClass=Auto  FilterContinuousStateAttributes=''  FilterStateMustResolveToSignalObject=off  FilterRTWStateStorageClass=Auto  ParallelPVariant=InternalParameters  IdealPVariant=Disabled  IVariant=InternalParameters  DVariant=Disabled  IntegratorVariant=Discrete  SatVariant=Disabled  AWVariant=Passthrough  PCopyVariant=Disabled  TRVariant=Disabled  FdbkBlocksVariant=Forward  IdealPFdbkVariant=Disabled  SatFdbkVariant=Disabled  DerivativeFilterVariant=Disabled  NVariant=Disabled  NCopyVariant=Disabled_SignalSpec  FilterICVariant=Disabled  IntegratorICVariant=InternalICs  ExternalResetVariant=Disabled  TRSumVariant=Passthrough  SumFdbkVariant=Disabled  SumVariant=Sum_PI  TsampFilterVariant=InternalTs  TsampNgainVariant=Passthrough  TsampIntegralVariant=Disabled_SignalSpec  ExternalSaturationOutDataTypeStr=Inherit: Same as second input  DerivativeSourceVariant=Disabled
  PID Controller3 : slpidlib/PID Controller  Controller=PI  Form=Parallel  TimeDomain=Discrete-time  UseExternalTs=off  SampleTime=-1  IntegratorMethod=Forward Euler  FilterMethod=Forward Euler  ControllerParametersSource=internal  P=1  I=500  UseKiTs=off  D=0  UseExternalDerivativeSource=off  N=100  UseFilter=on  TunerSelectOption=Transfer Function Based (PID Tuner App)  InitialConditionSource=internal  InitialConditionForIntegrator=0  InitialConditionForFilter=0  DifferentiatorICPrevScaledInput=0  ExternalReset=none  TrackingMode=off  Kt=1  LimitOutput=off  SatLimitsSource=internal  UpperSaturationLimit=inf  LowerSaturationLimit=-inf  LinearizeAsGain=on  AntiWindupMode=none  Kb=1  LimitIntegrator=off  UpperIntegratorSaturationLimit=inf  LowerIntegratorSaturationLimit=-inf  POutMin=[]  POutMax=[]  IOutMin=[]  IOutMax=[]  DOutMin=[]  DOutMax=[]  NOutMin=[]  NOutMax=[]  SumOutMin=[]  SumOutMax=[]  SaturationOutMin=[]  SaturationOutMax=[]  PParamMin=[]  PParamMax=[]  IParamMin=[]  IParamMax=[]  DParamMin=[]  DParamMax=[]  NParamMin=[]  NParamMax=[]  KbParamMin=[]  KbParamMax=[]  KtParamMin=[]  KtParamMax=[]  KbOutMin=[]  KbOutMax=[]  KtOutMin=[]  KtOutMax=[]  IntegratorOutMin=[]  IntegratorOutMax=[]  FilterOutMin=[]  FilterOutMax=[]  SumI1OutMin=[]  SumI1OutMax=[]  SumI2OutMin=[]  SumI2OutMax=[]  SumI3OutMin=[]  SumI3OutMax=[]  SumI4OutMin=[]  SumI4OutMax=[]  SumDOutMin=[]  SumDOutMax=[]  DifferentiatorOutMin=[]  DifferentiatorOutMax=[]  FilterDiffOutCoefMin=[]  FilterDiffOutCoefMax=[]  ReciprocalOutMin=[]  ReciprocalOutMax=[]  SumDenOutMin=[]  SumDenOutMax=[]  SumNumOutMin=[]  SumNumOutMax=[]  DivideOutMin=[]  DivideOutMax=[]  UdiffTsProdOutMin=[]  UdiffTsProdOutMax=[]  NTsProdOutMin=[]  NTsProdOutMax=[]  UintegralTsProdOutMin=[]  UintegralTsProdOutMax=[]  UngainTsProdOutMin=[]  UngainTsProdOutMax=[]  ClampingZeroOutDataTypeStr=Inherit: Inherit via back propagation  ClampingZeroOutMin=[]  ClampingZeroOutMax=[]  FilterDenConstantOutDataTypeStr=Inherit: Inherit via back propagation  FilterDenConstantOutMin=[]  FilterDenConstantOutMax=[]  PCopyOutDataTypeStr=Inherit: Inherit via back propagation  PCopyOutMin=[]  PCopyOutMax=[]  NCopyOutDataTypeStr=Inherit: Inherit via back propagation  NCopyOutMin=[]  NCopyOutMax=[]  IntegratorContinuousStateAttributes=''  IntegratorStateMustResolveToSignalObject=off  IntegratorRTWStateStorageClass=Auto  FilterContinuousStateAttributes=''  FilterStateMustResolveToSignalObject=off  FilterRTWStateStorageClass=Auto  ParallelPVariant=InternalParameters  IdealPVariant=Disabled  IVariant=InternalParameters  DVariant=Disabled  IntegratorVariant=Discrete  SatVariant=Disabled  AWVariant=Passthrough  PCopyVariant=Disabled  TRVariant=Disabled  FdbkBlocksVariant=Forward  IdealPFdbkVariant=Disabled  SatFdbkVariant=Disabled  DerivativeFilterVariant=Disabled  NVariant=Disabled  NCopyVariant=Disabled_SignalSpec  FilterICVariant=Disabled  IntegratorICVariant=InternalICs  ExternalResetVariant=Disabled  TRSumVariant=Passthrough  SumFdbkVariant=Disabled  SumVariant=Sum_PI  TsampFilterVariant=InternalTs  TsampNgainVariant=Passthrough  TsampIntegralVariant=Disabled_SignalSpec  ExternalSaturationOutDataTypeStr=Inherit: Same as second input  DerivativeSourceVariant=Disabled
  PLL (3ph) : spsPLL3phLib/PLL (3ph)  Fmin=45  Par_Init=[0, 50]  ParK=[180, 3200, 1]  TcD=1e-4  MaxRateChangeFreq=12  FilterCutOffFreq=25  Ts=50e-6  AGC=on
  PWM Generator (2-Level) : spsPWMGenerator2LevelLib/PWM Generator (2-Level)  ModulatorType=Three-phase bridge (6 pulses)  ModulatorMode=Unsynchronized  Fc=20e3  Pc=90  nF=27  MinMax="[ -1  1 ]"  SamplingTechnique=Natural  ModulatingSignals=off  m=0.8  Freq=50  Phase=0  Ts=50e-6  ShowCarrierOutport=off
  Vdc_ref : Constant  Value=730
  abc to dq0 : spsabctodq0Lib/abc to dq0  Alignment=90 degrees behind phase A axis
  abc to dq1 : spsabctodq0Lib/abc to dq0  Alignment=90 degrees behind phase A axis
  dq0 to abc : spsdq0toabcLib/dq0 to abc  Alignment=90 degrees behind phase A axis
  G : Outport
  wires:
  Vdc_ref/1 -> Add/1
  [Vdc] -> Add/2
  Add1/1 -> PID Controller1/1
  PID Controller1/1 -> Add2/1
  Add2/1 -> Add3/1
  Add3/1 -> Gain/1
  abc to dq0/1 -> Demux/1
  [Viabc] -> PLL (3ph)/1, abc to dq0/1
  PLL (3ph)/2 -> dq0 to abc/2, abc to dq1/2, abc to dq0/2
  [Iiabc] -> abc to dq1/1
  abc to dq1/1 -> Demux1/1
  Add5/1 -> Add7/1
  PID Controller2/1 -> Add5/1
  Add4/1 -> PID Controller2/1
  Demux1/2 -> Add4/2, Add2/2
  Iq_ref/1 -> Add4/1
  Demux/1 -> Add3/2
  Demux1/1 -> Add5/2, Add1/2
  Add7/1 -> Gain1/1
  Demux/2 -> Add7/2
  Gain/1 -> Mux/1
  Mux/1 -> dq0 to abc/1
  Gain1/1 -> Mux/2
  dq0 to abc/1 -> PWM Generator (2-Level)/1
  PWM Generator (2-Level)/1 -> G/1
  PID Controller3/1 -> Add1/1
  Add/1 -> PID Controller3/1

== system Fig_11_12_13_/PV ARRAY ==
  Irr (W/m²) : Inport
  Temp (°C) : Inport  Port=2
  Current Measurement : spsCurrentMeasurementLib/Current Measurement  PhasorSimulation=off  OutputType=Complex  PSBequivalent=0
  SOLAR PANEL 1 KW : spsPVArrayLib/PV Array  Npar=44  Nser=18  PlotType=array @ 1000 W/m2 & specified temperatures  S_vec="[ 1000  500  100 ]"  Temp_C_vec="[ 45 25  ]"  ModuleName=User-defined  PlotWhenSelected=off  Pm=214.6493  Ncell=60  Voc=36.3  Isc=7.84  Vm=29  Im=7.4017  beta_Voc_pc=-0.36099  alpha_Isc_pc=0.102  beta_Voc=-0.13104  alpha_Isc=0.0079968  IL=7.9095  I0=2.9374e-10  nI=0.98114  Rsh=294.0158  Rs=0.39142  RobustModel=off  RobustCellTemperature=313.3991  BAL=on  Tc=1e-6  Tfilter=5e-5
  T : Terminator
  Voltage Measurement : spsVoltageMeasurementLib/Voltage Measurement  PhasorSimulation=off  OutputType=Complex  PSBequivalent=0
  + : PMIOPort  Side=Right
  - : PMIOPort  Port=2  Side=Right
  tag scope: Ipv=global, Vpv=global
  wires:
  Voltage Measurement/1 -> [Vpv]
  Current Measurement/1 -> [Ipv]
  SOLAR PANEL 1 KW/1 -> T/1
  Irr (W/m²)/1 -> SOLAR PANEL 1 KW/1
  Temp (°C)/1 -> SOLAR PANEL 1 KW/2
  connections:
  Current Measurement/RConn1 -- +/RConn1 -- Voltage Measurement/LConn1
  Voltage Measurement/LConn2 -- -/RConn1 -- SOLAR PANEL 1 KW/RConn2
  SOLAR PANEL 1 KW/RConn1 -- Current Measurement/LConn1

== system Fig_11_12_13_/RESULTS ==
  RMS : spsRMSLib/RMS  TrueRMS=on  Freq=50  RMSInit=0  Ts=50e-6
  Scope1 : Scope
  Scope2 : Scope  NumInputPorts=3
  Scope3 : Scope
  wires:
  RMS/1 -> Scope1/1  "Rms"
  [Vlabc] -> Scope3/1, RMS/1  "Vlabc"
  [Vev] -> Scope2/3  "Vev"
  [Iev] -> Scope2/2  "Iev"
  [SOCbat] -> Scope2/1  "Soc"

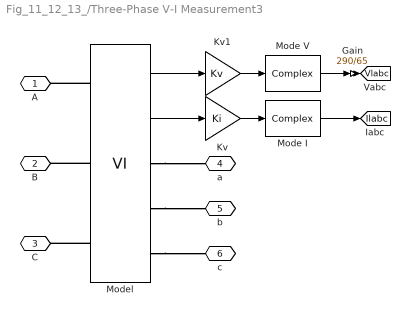
== system Fig_11_12_13_/Three-Phase V-I Measurement3 ==
  Gain : Gain  Gain=290/65
  Kv : Gain  Gain=Ki  SaturateOnIntegerOverflow=on  OutDataTypeStr=Inherit: Same as input  ParamDataTypeStr=Inherit: Same as input
  Kv1 : Gain  Gain=Kv  SaturateOnIntegerOverflow=on  OutDataTypeStr=Inherit: Same as input  ParamDataTypeStr=Inherit: Same as input
  Mode I : spsVIMeasurementModel/Complex  SystemSampleTime=-1  VariantActivationTime=update diagram  AllowFlexibleInterface=on  Latency=0  AutoFrameSizeCalculation=off
  Mode V : spsVIMeasurementModel/Complex  SystemSampleTime=-1  VariantActivationTime=update diagram  AllowFlexibleInterface=on  Latency=0  AutoFrameSizeCalculation=off
  Model : spsVIMeasurementModel/VI  SystemSampleTime=-1  VariantActivationTime=update diagram  AllowFlexibleInterface=on  Latency=0  AutoFrameSizeCalculation=off
  A : PMIOPort  Side=Left
  B : PMIOPort  Port=2  Side=Left
  C : PMIOPort  Port=3  Side=Left
  a : PMIOPort  Port=4  Side=Right
  b : PMIOPort  Port=5  Side=Right
  c : PMIOPort  Port=6  Side=Right
  tag scope: Ilabc=global, Vlabc=global
  wires:
  Mode V/1 -> Gain/1
  Mode I/1 -> [Ilabc]
  Kv1/1 -> Mode V/1
  Kv/1 -> Mode I/1
  Model/1 -> Kv1/1
  Model/2 -> Kv/1
  Gain/1 -> [Vlabc]
  connections:
  Model/LConn2 -- B/RConn1
  Model/LConn1 -- A/RConn1
  Model/LConn3 -- C/RConn1
  Model/RConn2 -- b/RConn1
  Model/RConn1 -- a/RConn1
  Model/RConn3 -- c/RConn1

== system Fig_11_12_13_/Variable Loads ==
  Three-Phase Series RLC Load2 : spsThreePhaseSeriesRLCLoadLib/Three-Phase Series RLC Load  LConnTagsString=A|B|C  Configuration=Y (grounded)  NominalVoltage=400  Vabc=[1e3 1e3 1e3]  Vabcp=[1e3 1e3 1e3]  NominalFrequency=50  UnbalancedPower=off  ActivePower=20e3  InductivePower=0  CapacitivePower=0  Pabc=[10e3 9e3 11e3]  QLabc=[100 90 110]  QCabc=[100 90 110]  Pabcp=[10e3 9e3 11e3]  QLabcp=[100 90 110]  QCabcp=[100 90 110]  Measurements=None  LoadType=constant Z
  Three-Phase Series RLC Load3 : spsThreePhaseSeriesRLCLoadLib/Three-Phase Series RLC Load  LConnTagsString=A|B|C  Configuration=Y (grounded)  NominalVoltage=400  Vabc=[1e3 1e3 1e3]  Vabcp=[1e3 1e3 1e3]  NominalFrequency=50  UnbalancedPower=off  ActivePower=20e3  InductivePower=0  CapacitivePower=0  Pabc=[10e3 9e3 11e3]  QLabc=[100 90 110]  QCabc=[100 90 110]  Pabcp=[10e3 9e3 11e3]  QLabcp=[100 90 110]  QCabcp=[100 90 110]  Measurements=None  LoadType=constant Z
  Three-Phase Breaker2 : spsThreePhaseBreakerLib/Three-Phase Breaker  InitialState=open  SwitchA=on  SwitchB=on  SwitchC=on  SwitchTimes=[0.2 0.4]  External=off  BreakerResistance=0.01  SnubberResistance=1e6  SnubberCapacitance=inf  Measurements=None
  Three-Phase Breaker3 : spsThreePhaseBreakerLib/Three-Phase Breaker  InitialState=closed  SwitchA=on  SwitchB=on  SwitchC=on  SwitchTimes=[0.6 0.8]  External=off  BreakerResistance=0.01  SnubberResistance=1e6  SnubberCapacitance=inf  Measurements=None
  a : PMIOPort  Side=Left
  b : PMIOPort  Port=2  Side=Left
  c : PMIOPort  Port=3  Side=Left
  connections:
  Three-Phase Breaker3/LConn2 -- Three-Phase Series RLC Load3/LConn2
  Three-Phase Breaker3/LConn1 -- Three-Phase Series RLC Load3/LConn1
  Three-Phase Breaker3/RConn3 -- Three-Phase Breaker2/RConn3 -- c/RConn1
  Three-Phase Breaker2/LConn1 -- Three-Phase Series RLC Load2/LConn1
  Three-Phase Breaker3/RConn1 -- a/RConn1 -- Three-Phase Breaker2/RConn1
  Three-Phase Breaker3/RConn2 -- Three-Phase Breaker2/RConn2 -- b/RConn1
  Three-Phase Breaker3/LConn3 -- Three-Phase Series RLC Load3/LConn3
  Three-Phase Breaker2/LConn2 -- Three-Phase Series RLC Load2/LConn2
  Three-Phase Breaker2/LConn3 -- Three-Phase Series RLC Load2/LConn3

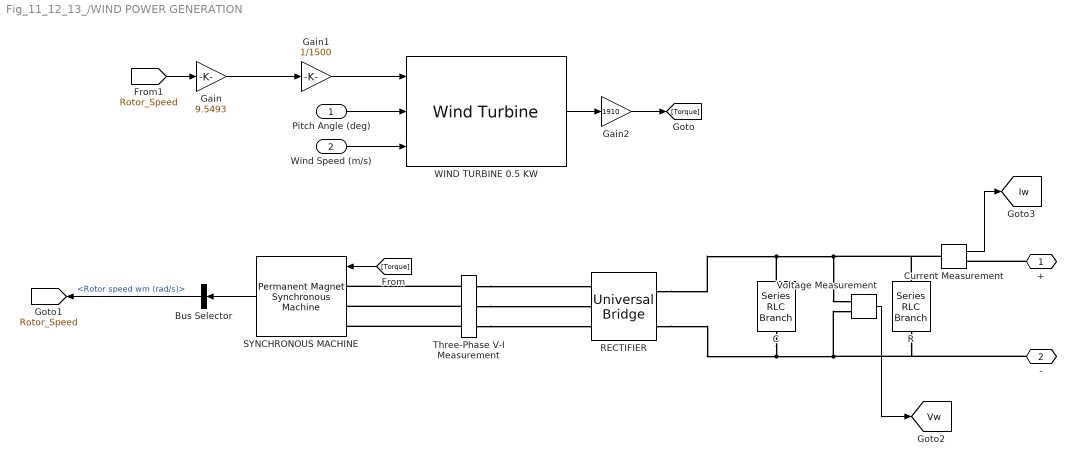
== system Fig_11_12_13_/WIND POWER GENERATION ==
  Pitch Angle (deg) : Inport
  Wind Speed (m/s) : Inport  Port=2
  Bus Selector : BusSelector  OutputSignals=Rotor speed wm (rad/s)
  C : spsSeriesRLCBranchLib/Series RLC Branch  LConnTagsString=__new0  RConnTagsString=__new0  BranchType=C  Resistance=20  Inductance=1e-3  SetiL0=off  InitialCurrent=0  Capacitance=1000e-6  Setx0=off  InitialVoltage=0  Measurements=None
  Current Measurement : spsCurrentMeasurementLib/Current Measurement  PhasorSimulation=off  OutputType=Complex  PSBequivalent=0
  Gain : Gain  Gain=9.5493
  Gain1 : Gain  Gain=1/1500
  Gain2 : Gain  Gain=1910
  R : spsSeriesRLCBranchLib/Series RLC Branch  LConnTagsString=__new0  RConnTagsString=__new0  BranchType=R  Resistance=15  Inductance=1e-3  SetiL0=off  InitialCurrent=0  Capacitance=10e-3  Setx0=off  InitialVoltage=0  Measurements=None
  RECTIFIER : spsUniversalBridgeLib/Universal Bridge  Arms=3  SnubberResistance=1e5  SnubberCapacitance=inf  Device=Diodes  Ron=1e-3  Lon=0  ForwardVoltages="[  0  0  ]"  ForwardVoltage=0  GTOparameters=[ 10e-6 , 20e-6 ]  IGBTparameters=[ 1e-6 , 2e-6 ]  Measurements=None  Measurements_2=None  converterType=Rectifier
  SYNCHRONOUS MACHINE : spsPermanentMagnetSynchronousMachineLib/Permanent Magnet Synchronous Machine  NbPhases=3  FluxDistribution=Sinusoidal  RotorType=Round  MechanicalLoad=Torque Tm  PresetModel=No  ShowDetailedParameters=on  MeasurementBus=off  Resistance=0.0485  Inductance=8.5e-3  dqInductances=[8.5e-3,8.5e-3]  La=0.000395  MachineConstant=Flux linkage established by magnets (V.s)  Flux=1.2  VoltageCst=870.6237  TorqueCst=7.2  Flat=120  Mechanical=[0.0027 0.0004924 4 0]  PolePairs=4  InitialConditions=[0,0, 0,0]  InitialConditions5ph=[0 0 0 0 0 0]  RefAngle=90 degrees behind phase A axis (modified Park)  IterativeDiscreteModel=Trapezoidal non iterative  TsBlock=50e-6  TsPowergui=0
  Three-Phase V-I Measurement : spsThreePhaseVIMeasurementLib/Three-Phase V-I Measurement  VoltageMeasurement=phase-to-phase  SetLabelV=on  LabelV=Vabc  Vpu=off  VpuLL=off  CurrentMeasurement=yes  SetLabelI=on  LabelI=Iabc  Ipu=off  Pbase=100e6  Vbase=500e3  OutputType=Complex  PhasorSimulation=off  PSBequivalent=0
  Voltage Measurement : spsVoltageMeasurementLib/Voltage Measurement  PhasorSimulation=off  OutputType=Complex  PSBequivalent=0
  WIND TURBINE 0.5 KW : spsWindTurbineLib/Wind Turbine  Pnom=300e3  Pelec_base=300e3/0.9  wind_base=12  P_wind_base=0.73  speed_nom=1.2  pitch_angle=0  c1_c6="[0.51763          116          0.4            5           21     0.006795]"  cp_nom=0.48  lambda_nom=8.1
  + : PMIOPort  Side=Right
  - : PMIOPort  Port=2  Side=Right
  tag scope: Iw=global, Rotor_Speed=global, Vw=global
  wires:
  [Rotor_Speed] -> Gain/1
  WIND TURBINE 0.5 KW/1 -> Gain2/1
  Pitch Angle (deg)/1 -> WIND TURBINE 0.5 KW/2
  Wind Speed (m/s)/1 -> WIND TURBINE 0.5 KW/3
  [Torque] -> SYNCHRONOUS MACHINE/1
  Bus Selector/1 -> [Rotor_Speed]  "<Rotor speed wm (rad/s)>"
  SYNCHRONOUS MACHINE/1 -> Bus Selector/1
  Gain/1 -> Gain1/1
  Gain1/1 -> WIND TURBINE 0.5 KW/1
  Gain2/1 -> [Torque]
  Voltage Measurement/1 -> [Vw]
  Current Measurement/1 -> [Iw]
  connections:
  C/RConn1 -- RECTIFIER/RConn2 -- Voltage Measurement/LConn2 -- -/RConn1 -- R/RConn1
  Three-Phase V-I Measurement/RConn1 -- RECTIFIER/LConn1
  Three-Phase V-I Measurement/LConn2 -- SYNCHRONOUS MACHINE/LConn2
  Three-Phase V-I Measurement/LConn3 -- SYNCHRONOUS MACHINE/LConn3
  Three-Phase V-I Measurement/RConn2 -- RECTIFIER/LConn2
  Three-Phase V-I Measurement/RConn3 -- RECTIFIER/LConn3
  Three-Phase V-I Measurement/LConn1 -- SYNCHRONOUS MACHINE/LConn1
  RECTIFIER/RConn1 -- C/LConn1 -- Voltage Measurement/LConn1 -- Current Measurement/LConn1 -- R/LConn1
  +/RConn1 -- Current Measurement/RConn1

== system Fig_11_12_13_/BOOST CONVERTER/PnO ==
  PERTURB & OBSERVE ALGORITHM : MATLAB Function  TreatAsAtomicUnit=on
  Saturation : Saturate  UpperLimit=0.2  LowerLimit=0.15
  D : Outport
  wires:
  [Vpv] -> PERTURB & OBSERVE ALGORITHM/1(Vpv)
  [Ipv] -> PERTURB & OBSERVE ALGORITHM/2(Ipv)
  PERTURB & OBSERVE ALGORITHM/1(D) -> Saturation/1
  Saturation/1 -> D/1

== system Fig_11_12_13_/BOOST CONVERTER1/PnO ==
  PERTURB & OBSERVE ALGORITHM : MATLAB Function  TreatAsAtomicUnit=on
  Saturation : Saturate  UpperLimit=1  LowerLimit=0
  D : Outport
  wires:
  [Vw] -> PERTURB & OBSERVE ALGORITHM/1(Vpv)
  [Iw] -> PERTURB & OBSERVE ALGORITHM/2(Ipv)
  PERTURB & OBSERVE ALGORITHM/1(D) -> Saturation/1
  Saturation/1 -> D/1

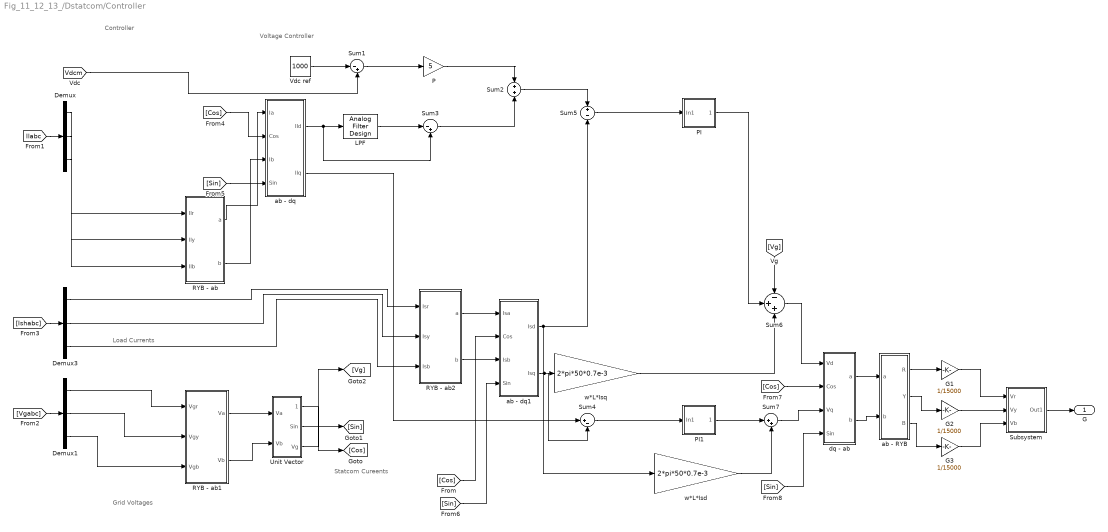
== system Fig_11_12_13_/Dstatcom/Controller ==
  note: Controller
  note: Voltage Controller
  note: Load Currents
  note: Grid Voltages
  note: Statcom Cureents
  Demux : Demux  Outputs=3
  Demux1 : Demux  Outputs=3
  Demux3 : Demux  Outputs=3
  G1 : Gain  Gain=1/15000
  G2 : Gain  Gain=1/15000
  G3 : Gain  Gain=1/15000
  LPF : dspfdesign/Analog Filter Design  method=Butterworth  filttype=Lowpass  N=5  Wlo=2*pi*50  Whi=80  Rp=2  Rs=40
  P : Gain  Gain=5
  PI : Subsystem
  PI1 : Subsystem
  RYB - ab : Subsystem
  RYB - ab1 : Subsystem
  RYB - ab2 : Subsystem
  Subsystem : Subsystem
  Sum1 : Sum  Inputs=|-+
  Sum2 : Sum
  Sum3 : Sum  Inputs=|-+
  Sum4 : Sum  Inputs=|+-
  Sum5 : Sum  Inputs=+-
  Sum6 : Sum  Inputs=-++
  Sum7 : Sum  Inputs=|++
  Unit Vector : Subsystem
  Vdc ref : Constant  Value=1000
  ab - RYB : Subsystem
  ab - dq : Subsystem
  ab - dq1 : Subsystem
  dq - ab : Subsystem
  w*L*Isd : Gain  Gain=2*pi*50*0.7e-3
  w*L*Isq : Gain  Gain=2*pi*50*0.7e-3
  G : Outport
  wires:
  Vdc ref/1 -> Sum1/1
  [Cos] -> ab - dq/2(Cos)
  Sum2/1 -> Sum5/1
  RYB - ab/1(a) -> ab - dq/1(Ia)
  RYB - ab/2(b) -> ab - dq/3(Ib)
  Sum6/1 -> dq - ab/1(Vd)
  [Sin] -> ab - dq/4(Sin)
  dq - ab/1(a) -> ab - RYB/1(a)
  RYB - ab1/1(Va) -> Unit Vector/1(Va)
  RYB - ab1/2(Vb) -> Unit Vector/2(Vb)
  Subsystem/1(Out1) -> G/1
  [Cos] -> dq - ab/2(Cos)
  ab - dq/2(Ilq) -> Sum4/1
  ab - dq/1(Ild) -> Sum3/2, LPF/1
  Unit Vector/1(Cos) -> [Cos]
  [Ilabc] -> Demux/1
  Unit Vector/3(Vg) -> [Vg]
  Unit Vector/2(Sin) -> [Sin]
  Sum1/1 -> P/1
  LPF/1 -> Sum3/1
  P/1 -> Sum2/1
  w*L*Isd/1 -> Sum7/2
  [Sin] -> ab - dq1/4(Sin)
  Sum3/1 -> Sum2/2
  RYB - ab2/1(a) -> ab - dq1/1(Isa)
  RYB - ab2/2(b) -> ab - dq1/3(Isb)
  [Cos] -> ab - dq1/2(Cos)
  ab - dq1/1(Isd) -> Sum5/2, w*L*Isd/1
  PI/1(Out1) -> Sum6/2
  ab - dq1/2(Isq) -> Sum4/2, w*L*Isq/1
  [Sin] -> dq - ab/4(Sin)
  Sum5/1 -> PI/1(In1)
  w*L*Isq/1 -> Sum6/3
  [Vgabc] -> Demux1/1
  Sum4/1 -> PI1/1(In1)
  [Vg] -> Sum6/1
  PI1/1(Out1) -> Sum7/1
  Sum7/1 -> dq - ab/3(Vq)
  dq - ab/2(b) -> ab - RYB/2(b)
  ab - RYB/1(R) -> G1/1
  ab - RYB/3(B) -> G3/1
  ab - RYB/2(Y) -> G2/1
  Demux/3 -> RYB - ab/3(Ilb)
  [Ishabc] -> Demux3/1
  Demux/2 -> RYB - ab/2(Ily)
  Demux/1 -> RYB - ab/1(Ilr)
  G1/1 -> Subsystem/1(Vr)
  Demux1/1 -> RYB - ab1/1(Vgr)
  Demux3/2 -> RYB - ab2/2(Isy)
  Demux3/1 -> RYB - ab2/1(Isr)
  G2/1 -> Subsystem/2(Vy)
  G3/1 -> Subsystem/3(Vb)
  Demux3/3 -> RYB - ab2/3(Isb)
  [Vdcm] -> Sum1/2
  Demux1/3 -> RYB - ab1/3(Vgb)
  Demux1/2 -> RYB - ab1/2(Vgy)

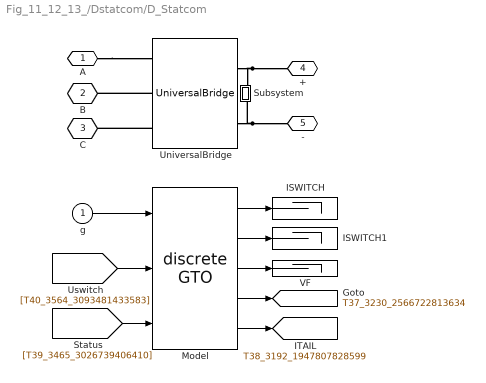
== system Fig_11_12_13_/Dstatcom/D_Statcom ==
  g : Inport
  ISWITCH : Terminator
  ISWITCH1 : Terminator
  Model : spsUniversalBridgeModel/discrete GTO  SystemSampleTime=-1  VariantActivationTime=update diagram  AllowFlexibleInterface=on  Latency=0  AutoFrameSizeCalculation=off
      settings: LibrarySourceBlock=spsUniversalBridgeModel/discrete IGBT
  Subsystem : Subsystem
      settings: PortSchema="{\"entries\":[{\"content\":{\"sides\":[{\"content\":{},\"type\":\"ConnectorPlacement.EquallySpacedRectSide\",\"uuid\":\"45ed6523-8129-430d-b695-ab779cead3b3\"},{\"content\":{\"side\":\"RIGHT\"},\"type\":\"ConnectorPlacement.EquallySpacedRectSide\",\"uuid\":\"0321dbd1-bfa6-4d12-9847-db0ab2db333c\"},{\"content\":{\"connectorIds\":[\"LConn1\"],\"side\":\"TOP\"},\"type\":\"ConnectorPlacement.EquallySpacedRectSide\",\"uuid\":\"d2f7f7f0-e5c6-4a13-80de-db08eddbc3d3\"},{\"content\":{\"connectorIds\":[\"RConn1\"],\"side\":\"BOTTOM\"},\"type\":\"ConnectorPlacement.EquallySpacedRectSide\",\"uuid\":\"69d13cc0-ae1f-4e4b-8477-de35a67103d6\"}]},\"type\":\"ConnectorPlacement.EquallySpacedConnector\",\"uuid\":\"761758ce-a32d-498f-9c9b-ff1ef3c8683f\"}],\"packageUris\":[\"http://schema.mathworks.com/mf0/Connector/R2020b\"],\"version\":\"1.0\"}"
  UniversalBridge : spsUniversalBridgeLib/Universal Bridge/UniversalBridge  PhysicalDomain=powersysdomain  SubClassName=unknown  LeftPortType=p1  RightPortType=p1  LConnTagsString=A|B|C  RConnTagsString=+|-
  VF : Terminator
  A : PMIOPort  Side=Left
  B : PMIOPort  Port=2  Side=Left
  C : PMIOPort  Port=3  Side=Left
  + : PMIOPort  Port=4  Side=Right
  - : PMIOPort  Port=5  Side=Right
  tag scope: T37_3230_2566722813634=global, T38_3192_1947807828599=global
  wires:
  Model/3 -> VF/1
  Model/1 -> ISWITCH/1
  [T39_3465_3026739406410] -> Model/3
  Model/2 -> ISWITCH1/1
  Model/4 -> [T37_3230_2566722813634]
  g/1 -> Model/1
  Model/5 -> [T38_3192_1947807828599]
  [T40_3564_3093481433583] -> Model/2
  connections:
  A/RConn1 -- UniversalBridge/LConn1
  UniversalBridge/RConn1 -- +/RConn1 -- Subsystem/LConn1
  UniversalBridge/LConn3 -- C/RConn1
  UniversalBridge/RConn2 -- -/RConn1 -- Subsystem/RConn1
  UniversalBridge/LConn2 -- B/RConn1
